simulink model "CoupledTanks_original"  (R2023b)
settings: Solver=ode45  StartTime=0.0  StopTime=400  MaxStep=1e-1  RelTol=1e-3  EnableMultiTasking=on
InitFcn:
  | g = 9.81; %gravitational constant
  | 
  | % showVR = 1; %show VR world
  | % h1_init = 0; %initial condition
  | % h2_init = 0; %initial condition
values from neighbouring files (symbols this model uses):
  K = place(Acl,Bcl, xd)    [ARI_SEM.m]
undefined symbols (not defined in the file or in its folder): P
libraries: vrlib x56, cstblocks x3, slpidlib x1
(part 2 of 2)

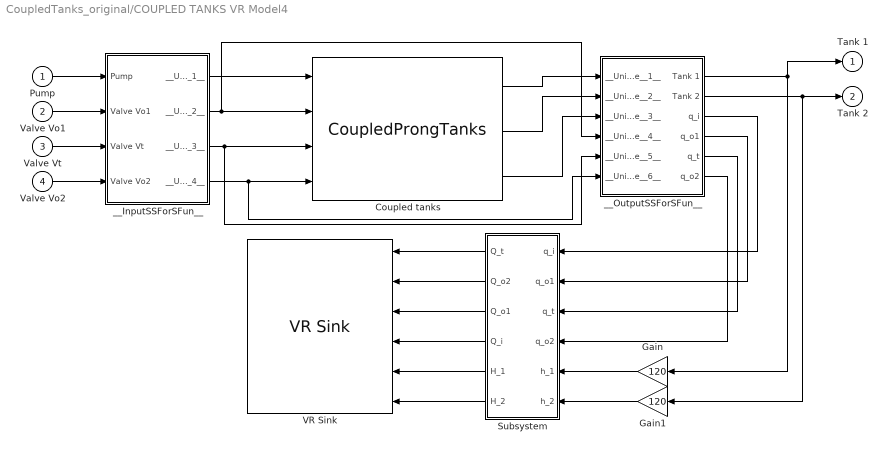
== system CoupledTanks_original/COUPLED TANKS VR Model4 ==
  Pump : Inport
  Valve Vo1 : Inport  Port=2
  Valve Vt : Inport  Port=3
  Valve Vo2 : Inport  Port=4
  Coupled tanks : M-S-Function  FunctionName=CoupledProngTanks  Parameters=h10 h20  mask{h10=sfcnParam1, h20=sfcnParam2}
      mask prompts: h10 "h1_init"; h20 "h2_init"
      mask Display:
      | port_label('input',1,'Pump');
      | port_label('input',2,'Valve Vo1');
      | port_label('input',3,'Valve Vt');
      | port_label('input',4,'Valve Vo2');
      | port_label('output',1,'Tank 1');
      | port_label('output',2,'Tank 2');
      | port_label('output',3,'q_i');
  Gain : Gain  Gain=120
  Gain1 : Gain  Gain=120
  Subsystem : Subsystem
  VR Sink : vrlib/VR Sink  InstantiateOnLoad=on  SampleTime=-1  ViewEnable=on  RemoteChange=off  RemoteView=on  FieldsWritten=Valve_t.rotation.4.1.double#Valve_o2.rotation.4.1.double#Valve_o1.rotation.4.1.double#Pump.rotation.4.1.double#water1.scale.3.1.double#water2.scale.3.1.double  WorldFileName=CoupledTanks_VR.WRL  AutoView=off  VideoDimensions=[]  AllowVariableSize=off
  __InputSSForSFun__ : Subsystem
  __OutputSSForSFun__ : Subsystem
  Tank 1 : Outport  OutDataTypeStr=double  PortDimensions=1  SampleTime=[-1 0]
  Tank 2 : Outport  Port=2  OutDataTypeStr=double  PortDimensions=1  SampleTime=[-1 0]
  wires:
  __OutputSSForSFun__/6(q_o2) -> Subsystem/4(q_o2)
  __OutputSSForSFun__/5(q_t) -> Subsystem/3(q_t)
  __OutputSSForSFun__/4(q_o1) -> Subsystem/2(q_o1)
  __OutputSSForSFun__/3(q_i) -> Subsystem/1(q_i)
  Subsystem/2(Q_o2) -> VR Sink/2
  Subsystem/3(Q_o1) -> VR Sink/3
  Subsystem/4(Q_i) -> VR Sink/4
  Subsystem/1(Q_t) -> VR Sink/1
  Subsystem/6(H_2) -> VR Sink/6
  Subsystem/5(H_1) -> VR Sink/5
  __OutputSSForSFun__/2(Tank 2) -> Gain1/1, Tank 2/1
  __OutputSSForSFun__/1(Tank 1) -> Tank 1/1, Gain/1
  __InputSSForSFun__/4(__UniqueOutportName__4__) -> __OutputSSForSFun__/6(__UniqueInportName__6__), Coupled tanks/4
  __InputSSForSFun__/3(__UniqueOutportName__3__) -> __OutputSSForSFun__/5(__UniqueInportName__5__), Coupled tanks/3
  Coupled tanks/2 -> __OutputSSForSFun__/2(__UniqueInportName__2__)
  Coupled tanks/1 -> __OutputSSForSFun__/1(__UniqueInportName__1__)
  __InputSSForSFun__/2(__UniqueOutportName__2__) -> __OutputSSForSFun__/4(__UniqueInportName__4__), Coupled tanks/2
  __InputSSForSFun__/1(__UniqueOutportName__1__) -> Coupled tanks/1
  Valve Vo2/1 -> __InputSSForSFun__/4(Valve Vo2)
  Valve Vt/1 -> __InputSSForSFun__/3(Valve Vt)
  Valve Vo1/1 -> __InputSSForSFun__/2(Valve Vo1)
  Pump/1 -> __InputSSForSFun__/1(Pump)
  Coupled tanks/3 -> __OutputSSForSFun__/3(__UniqueInportName__3__)
  Gain/1 -> Subsystem/5(h_1)
  Gain1/1 -> Subsystem/6(h_2)

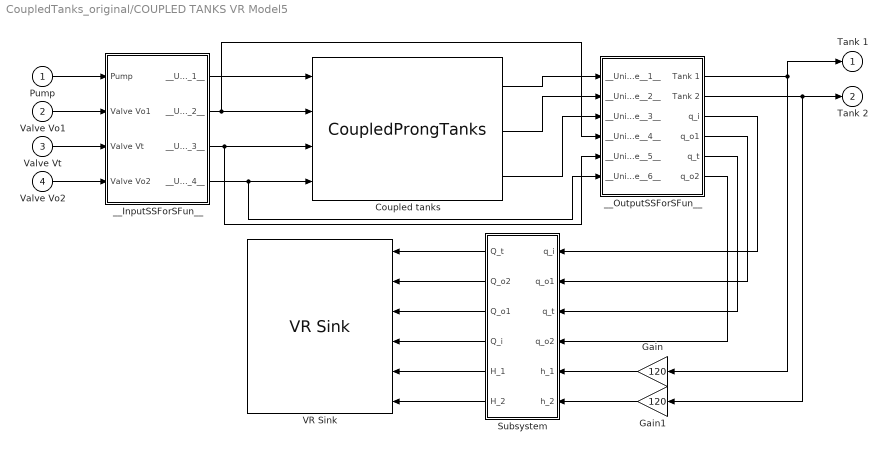
== system CoupledTanks_original/COUPLED TANKS VR Model5 ==
  Pump : Inport
  Valve Vo1 : Inport  Port=2
  Valve Vt : Inport  Port=3
  Valve Vo2 : Inport  Port=4
  Coupled tanks : M-S-Function  FunctionName=CoupledProngTanks  Parameters=h10 h20  mask{h10=sfcnParam1, h20=sfcnParam2}
      mask prompts: h10 "h1_init"; h20 "h2_init"
      mask Display:
      | port_label('input',1,'Pump');
      | port_label('input',2,'Valve Vo1');
      | port_label('input',3,'Valve Vt');
      | port_label('input',4,'Valve Vo2');
      | port_label('output',1,'Tank 1');
      | port_label('output',2,'Tank 2');
      | port_label('output',3,'q_i');
  Gain : Gain  Gain=120
  Gain1 : Gain  Gain=120
  Subsystem : Subsystem
  VR Sink : vrlib/VR Sink  InstantiateOnLoad=on  SampleTime=-1  ViewEnable=on  RemoteChange=off  RemoteView=on  FieldsWritten=Valve_t.rotation.4.1.double#Valve_o2.rotation.4.1.double#Valve_o1.rotation.4.1.double#Pump.rotation.4.1.double#water1.scale.3.1.double#water2.scale.3.1.double  WorldFileName=CoupledTanks_VR.WRL  AutoView=off  VideoDimensions=[]  AllowVariableSize=off
  __InputSSForSFun__ : Subsystem
  __OutputSSForSFun__ : Subsystem
  Tank 1 : Outport  OutDataTypeStr=double  PortDimensions=1  SampleTime=[-1 0]
  Tank 2 : Outport  Port=2  OutDataTypeStr=double  PortDimensions=1  SampleTime=[-1 0]
  wires:
  __OutputSSForSFun__/6(q_o2) -> Subsystem/4(q_o2)
  __OutputSSForSFun__/5(q_t) -> Subsystem/3(q_t)
  __OutputSSForSFun__/4(q_o1) -> Subsystem/2(q_o1)
  __OutputSSForSFun__/3(q_i) -> Subsystem/1(q_i)
  Subsystem/2(Q_o2) -> VR Sink/2
  Subsystem/3(Q_o1) -> VR Sink/3
  Subsystem/4(Q_i) -> VR Sink/4
  Subsystem/1(Q_t) -> VR Sink/1
  Subsystem/6(H_2) -> VR Sink/6
  Subsystem/5(H_1) -> VR Sink/5
  __OutputSSForSFun__/2(Tank 2) -> Gain1/1, Tank 2/1
  __OutputSSForSFun__/1(Tank 1) -> Tank 1/1, Gain/1
  __InputSSForSFun__/4(__UniqueOutportName__4__) -> __OutputSSForSFun__/6(__UniqueInportName__6__), Coupled tanks/4
  __InputSSForSFun__/3(__UniqueOutportName__3__) -> __OutputSSForSFun__/5(__UniqueInportName__5__), Coupled tanks/3
  Coupled tanks/2 -> __OutputSSForSFun__/2(__UniqueInportName__2__)
  Coupled tanks/1 -> __OutputSSForSFun__/1(__UniqueInportName__1__)
  __InputSSForSFun__/2(__UniqueOutportName__2__) -> __OutputSSForSFun__/4(__UniqueInportName__4__), Coupled tanks/2
  __InputSSForSFun__/1(__UniqueOutportName__1__) -> Coupled tanks/1
  Valve Vo2/1 -> __InputSSForSFun__/4(Valve Vo2)
  Valve Vt/1 -> __InputSSForSFun__/3(Valve Vt)
  Valve Vo1/1 -> __InputSSForSFun__/2(Valve Vo1)
  Pump/1 -> __InputSSForSFun__/1(Pump)
  Coupled tanks/3 -> __OutputSSForSFun__/3(__UniqueInportName__3__)
  Gain/1 -> Subsystem/5(h_1)
  Gain1/1 -> Subsystem/6(h_2)

== system CoupledTanks_original/COUPLED TANKS VR Model6 ==
  Pump : Inport
  Valve Vo1 : Inport  Port=2
  Valve Vt : Inport  Port=3
  Valve Vo2 : Inport  Port=4
  Coupled tanks : M-S-Function  FunctionName=CoupledProngTanks  Parameters=h10 h20  mask{h10=sfcnParam1, h20=sfcnParam2}
      mask prompts: h10 "h1_init"; h20 "h2_init"
      mask Display:
      | port_label('input',1,'Pump');
      | port_label('input',2,'Valve Vo1');
      | port_label('input',3,'Valve Vt');
      | port_label('input',4,'Valve Vo2');
      | port_label('output',1,'Tank 1');
      | port_label('output',2,'Tank 2');
      | port_label('output',3,'q_i');
  Subsystem : Subsystem
  VR Sink : vrlib/VR Sink  InstantiateOnLoad=on  SampleTime=-1  ViewEnable=on  RemoteChange=off  RemoteView=on  FieldsWritten=Valve_t.rotation.4.1.double#Valve_o2.rotation.4.1.double#Valve_o1.rotation.4.1.double#Pump.rotation.4.1.double#water1.scale.3.1.double#water2.scale.3.1.double  WorldFileName=CoupledTanks_VR.WRL  AutoView=off  VideoDimensions=[]  AllowVariableSize=off
  __InputSSForSFun__ : Subsystem
  __OutputSSForSFun__ : Subsystem
  Tank 1 : Outport  OutDataTypeStr=double  PortDimensions=1  SampleTime=[-1 0]
  Tank 2 : Outport  Port=2  OutDataTypeStr=double  PortDimensions=1  SampleTime=[-1 0]
  wires:
  __OutputSSForSFun__/6(q_o2) -> Subsystem/4(q_o2)
  __OutputSSForSFun__/5(q_t) -> Subsystem/3(q_t)
  __OutputSSForSFun__/4(q_o1) -> Subsystem/2(q_o1)
  __OutputSSForSFun__/3(q_i) -> Subsystem/1(q_i)
  Subsystem/2(Q_o2) -> VR Sink/2
  Subsystem/3(Q_o1) -> VR Sink/3
  Subsystem/4(Q_i) -> VR Sink/4
  Subsystem/1(Q_t) -> VR Sink/1
  Subsystem/6(H_2) -> VR Sink/6
  Subsystem/5(H_1) -> VR Sink/5
  __OutputSSForSFun__/2(Tank 2) -> Subsystem/6(h_2), Tank 2/1
  __OutputSSForSFun__/1(Tank 1) -> Tank 1/1, Subsystem/5(h_1)
  __InputSSForSFun__/4(__UniqueOutportName__4__) -> __OutputSSForSFun__/6(__UniqueInportName__6__), Coupled tanks/4
  __InputSSForSFun__/3(__UniqueOutportName__3__) -> __OutputSSForSFun__/5(__UniqueInportName__5__), Coupled tanks/3
  Coupled tanks/2 -> __OutputSSForSFun__/2(__UniqueInportName__2__)
  Coupled tanks/1 -> __OutputSSForSFun__/1(__UniqueInportName__1__)
  __InputSSForSFun__/2(__UniqueOutportName__2__) -> __OutputSSForSFun__/4(__UniqueInportName__4__), Coupled tanks/2
  __InputSSForSFun__/1(__UniqueOutportName__1__) -> Coupled tanks/1
  Valve Vo2/1 -> __InputSSForSFun__/4(Valve Vo2)
  Valve Vt/1 -> __InputSSForSFun__/3(Valve Vt)
  Valve Vo1/1 -> __InputSSForSFun__/2(Valve Vo1)
  Pump/1 -> __InputSSForSFun__/1(Pump)
  Coupled tanks/3 -> __OutputSSForSFun__/3(__UniqueInportName__3__)

== system CoupledTanks_original/COUPLED TANKS VR Model7 ==
  Pump : Inport
  Valve Vo1 : Inport  Port=2
  Valve Vt : Inport  Port=3
  Valve Vo2 : Inport  Port=4
  Coupled tanks : M-S-Function  FunctionName=CoupledProngTanks  Parameters=h10 h20  mask{h10=sfcnParam1, h20=sfcnParam2}
      mask prompts: h10 "h1_init"; h20 "h2_init"
      mask Display:
      | port_label('input',1,'Pump');
      | port_label('input',2,'Valve Vo1');
      | port_label('input',3,'Valve Vt');
      | port_label('input',4,'Valve Vo2');
      | port_label('output',1,'Tank 1');
      | port_label('output',2,'Tank 2');
      | port_label('output',3,'q_i');
  Gain : Gain  Gain=120
  Gain1 : Gain  Gain=120
  Subsystem : Subsystem
  VR Sink : vrlib/VR Sink  InstantiateOnLoad=on  SampleTime=-1  ViewEnable=on  RemoteChange=off  RemoteView=on  FieldsWritten=Valve_t.rotation.4.1.double#Valve_o2.rotation.4.1.double#Valve_o1.rotation.4.1.double#Pump.rotation.4.1.double#water1.scale.3.1.double#water2.scale.3.1.double  WorldFileName=CoupledTanks_VR.WRL  AutoView=off  VideoDimensions=[]  AllowVariableSize=off
  __InputSSForSFun__ : Subsystem
  __OutputSSForSFun__ : Subsystem
  Tank 1 : Outport  OutDataTypeStr=double  PortDimensions=1  SampleTime=[-1 0]
  Tank 2 : Outport  Port=2  OutDataTypeStr=double  PortDimensions=1  SampleTime=[-1 0]
  wires:
  __OutputSSForSFun__/6(q_o2) -> Subsystem/4(q_o2)
  __OutputSSForSFun__/5(q_t) -> Subsystem/3(q_t)
  __OutputSSForSFun__/4(q_o1) -> Subsystem/2(q_o1)
  __OutputSSForSFun__/3(q_i) -> Subsystem/1(q_i)
  Subsystem/2(Q_o2) -> VR Sink/2
  Subsystem/3(Q_o1) -> VR Sink/3
  Subsystem/4(Q_i) -> VR Sink/4
  Subsystem/1(Q_t) -> VR Sink/1
  Subsystem/6(H_2) -> VR Sink/6
  Subsystem/5(H_1) -> VR Sink/5
  __OutputSSForSFun__/2(Tank 2) -> Gain1/1, Tank 2/1
  __OutputSSForSFun__/1(Tank 1) -> Tank 1/1, Gain/1
  __InputSSForSFun__/4(__UniqueOutportName__4__) -> __OutputSSForSFun__/6(__UniqueInportName__6__), Coupled tanks/4
  __InputSSForSFun__/3(__UniqueOutportName__3__) -> __OutputSSForSFun__/5(__UniqueInportName__5__), Coupled tanks/3
  Coupled tanks/2 -> __OutputSSForSFun__/2(__UniqueInportName__2__)
  Coupled tanks/1 -> __OutputSSForSFun__/1(__UniqueInportName__1__)
  __InputSSForSFun__/2(__UniqueOutportName__2__) -> __OutputSSForSFun__/4(__UniqueInportName__4__), Coupled tanks/2
  __InputSSForSFun__/1(__UniqueOutportName__1__) -> Coupled tanks/1
  Valve Vo2/1 -> __InputSSForSFun__/4(Valve Vo2)
  Valve Vt/1 -> __InputSSForSFun__/3(Valve Vt)
  Valve Vo1/1 -> __InputSSForSFun__/2(Valve Vo1)
  Pump/1 -> __InputSSForSFun__/1(Pump)
  Coupled tanks/3 -> __OutputSSForSFun__/3(__UniqueInportName__3__)
  Gain/1 -> Subsystem/5(h_1)
  Gain1/1 -> Subsystem/6(h_2)

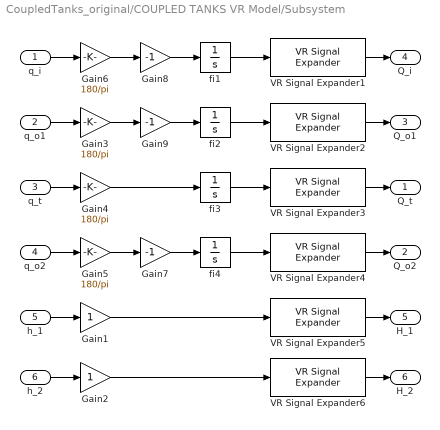
== system CoupledTanks_original/COUPLED TANKS VR Model/Subsystem ==
  q_i : Inport
  q_o1 : Inport  Port=2
  q_t : Inport  Port=3
  q_o2 : Inport  Port=4
  h_1 : Inport  Port=5
  h_2 : Inport  Port=6
  Gain1 : Gain
  Gain2 : Gain
  Gain{3..6} (4 alike) : Gain  Gain=180/pi
  Gain7 : Gain  Gain=-1
  Gain8 : Gain  Gain=-1
  Gain9 : Gain  Gain=-1
  VR Signal Expander{1..4} (4 alike) : vrlib/VR Signal Expander  outwidth=4  outidx=[4]
  VR Signal Expander5 : vrlib/VR Signal Expander  outwidth=3  outidx=[2]
  VR Signal Expander6 : vrlib/VR Signal Expander  outwidth=3  outidx=[2]
  fi{1..4} (4 alike) : Integrator
  Q_t : Outport
  Q_o2 : Outport  Port=2
  Q_o1 : Outport  Port=3
  Q_i : Outport  Port=4
  H_1 : Outport  Port=5
  H_2 : Outport  Port=6
  wires:
  Gain9/1 -> fi2/1
  Gain8/1 -> fi1/1
  Gain7/1 -> fi4/1
  Gain5/1 -> Gain7/1
  q_o2/1 -> Gain5/1
  VR Signal Expander4/1 -> Q_o2/1
  fi4/1 -> VR Signal Expander4/1
  Gain4/1 -> fi3/1
  Gain6/1 -> Gain8/1
  Gain3/1 -> Gain9/1
  q_t/1 -> Gain4/1
  q_o1/1 -> Gain3/1
  Gain2/1 -> VR Signal Expander6/1
  Gain1/1 -> VR Signal Expander5/1
  VR Signal Expander6/1 -> H_2/1
  VR Signal Expander5/1 -> H_1/1
  VR Signal Expander1/1 -> Q_i/1
  VR Signal Expander2/1 -> Q_o1/1
  VR Signal Expander3/1 -> Q_t/1
  h_2/1 -> Gain2/1
  h_1/1 -> Gain1/1
  q_i/1 -> Gain6/1
  fi2/1 -> VR Signal Expander2/1
  fi3/1 -> VR Signal Expander3/1
  fi1/1 -> VR Signal Expander1/1

== system CoupledTanks_original/COUPLED TANKS VR Model/__InputSSForSFun__ ==
  Pump : Inport
  Valve Vo1 : Inport  Port=2
  Valve Vt : Inport  Port=3
  Valve Vo2 : Inport  Port=4
  __UniqueOutportName__1__ : Outport
  __UniqueOutportName__2__ : Outport  Port=2
  __UniqueOutportName__3__ : Outport  Port=3
  __UniqueOutportName__4__ : Outport  Port=4
  wires:
  Valve Vo2/1 -> __UniqueOutportName__4__/1
  Valve Vt/1 -> __UniqueOutportName__3__/1
  Valve Vo1/1 -> __UniqueOutportName__2__/1
  Pump/1 -> __UniqueOutportName__1__/1

== system CoupledTanks_original/COUPLED TANKS VR Model/__OutputSSForSFun__ ==
  __UniqueInportName__1__ : Inport
  __UniqueInportName__2__ : Inport  Port=2
  __UniqueInportName__3__ : Inport  Port=3
  __UniqueInportName__4__ : Inport  Port=4
  __UniqueInportName__5__ : Inport  Port=5
  __UniqueInportName__6__ : Inport  Port=6
  Tank 1 : Outport  OutDataTypeStr=double  PortDimensions=1  SampleTime=[-1 0]
  Tank 2 : Outport  Port=2  OutDataTypeStr=double  PortDimensions=1  SampleTime=[-1 0]
  q_i : Outport  Port=3  OutDataTypeStr=double  PortDimensions=1  SampleTime=[0 1]
  q_o1 : Outport  Port=4  OutDataTypeStr=double  PortDimensions=1  SampleTime=[-1 0]
  q_t : Outport  Port=5  OutDataTypeStr=double  PortDimensions=1  SampleTime=[-1 0]
  q_o2 : Outport  Port=6  OutDataTypeStr=double  PortDimensions=1  SampleTime=[-1 0]
  wires:
  __UniqueInportName__6__/1 -> q_o2/1
  __UniqueInportName__5__/1 -> q_t/1
  __UniqueInportName__4__/1 -> q_o1/1
  __UniqueInportName__3__/1 -> q_i/1
  __UniqueInportName__2__/1 -> Tank 2/1
  __UniqueInportName__1__/1 -> Tank 1/1

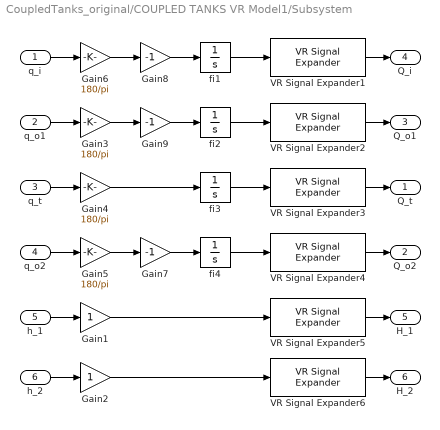
== system CoupledTanks_original/COUPLED TANKS VR Model1/Subsystem ==
  q_i : Inport
  q_o1 : Inport  Port=2
  q_t : Inport  Port=3
  q_o2 : Inport  Port=4
  h_1 : Inport  Port=5
  h_2 : Inport  Port=6
  Gain1 : Gain
  Gain2 : Gain
  Gain{3..6} (4 alike) : Gain  Gain=180/pi
  Gain7 : Gain  Gain=-1
  Gain8 : Gain  Gain=-1
  Gain9 : Gain  Gain=-1
  VR Signal Expander{1..4} (4 alike) : vrlib/VR Signal Expander  outwidth=4  outidx=[4]
  VR Signal Expander5 : vrlib/VR Signal Expander  outwidth=3  outidx=[2]
  VR Signal Expander6 : vrlib/VR Signal Expander  outwidth=3  outidx=[2]
  fi{1..4} (4 alike) : Integrator
  Q_t : Outport
  Q_o2 : Outport  Port=2
  Q_o1 : Outport  Port=3
  Q_i : Outport  Port=4
  H_1 : Outport  Port=5
  H_2 : Outport  Port=6
  wires:
  Gain9/1 -> fi2/1
  Gain8/1 -> fi1/1
  Gain7/1 -> fi4/1
  Gain5/1 -> Gain7/1
  q_o2/1 -> Gain5/1
  VR Signal Expander4/1 -> Q_o2/1
  fi4/1 -> VR Signal Expander4/1
  Gain4/1 -> fi3/1
  Gain6/1 -> Gain8/1
  Gain3/1 -> Gain9/1
  q_t/1 -> Gain4/1
  q_o1/1 -> Gain3/1
  Gain2/1 -> VR Signal Expander6/1
  Gain1/1 -> VR Signal Expander5/1
  VR Signal Expander6/1 -> H_2/1
  VR Signal Expander5/1 -> H_1/1
  VR Signal Expander1/1 -> Q_i/1
  VR Signal Expander2/1 -> Q_o1/1
  VR Signal Expander3/1 -> Q_t/1
  h_2/1 -> Gain2/1
  h_1/1 -> Gain1/1
  q_i/1 -> Gain6/1
  fi2/1 -> VR Signal Expander2/1
  fi3/1 -> VR Signal Expander3/1
  fi1/1 -> VR Signal Expander1/1

== system CoupledTanks_original/COUPLED TANKS VR Model1/__InputSSForSFun__ ==
  Pump : Inport
  Valve Vo1 : Inport  Port=2
  Valve Vt : Inport  Port=3
  Valve Vo2 : Inport  Port=4
  __UniqueOutportName__1__ : Outport
  __UniqueOutportName__2__ : Outport  Port=2
  __UniqueOutportName__3__ : Outport  Port=3
  __UniqueOutportName__4__ : Outport  Port=4
  wires:
  Valve Vo2/1 -> __UniqueOutportName__4__/1
  Valve Vt/1 -> __UniqueOutportName__3__/1
  Valve Vo1/1 -> __UniqueOutportName__2__/1
  Pump/1 -> __UniqueOutportName__1__/1

== system CoupledTanks_original/COUPLED TANKS VR Model1/__OutputSSForSFun__ ==
  __UniqueInportName__1__ : Inport
  __UniqueInportName__2__ : Inport  Port=2
  __UniqueInportName__3__ : Inport  Port=3
  __UniqueInportName__4__ : Inport  Port=4
  __UniqueInportName__5__ : Inport  Port=5
  __UniqueInportName__6__ : Inport  Port=6
  Tank 1 : Outport  OutDataTypeStr=double  PortDimensions=1  SampleTime=[-1 0]
  Tank 2 : Outport  Port=2  OutDataTypeStr=double  PortDimensions=1  SampleTime=[-1 0]
  q_i : Outport  Port=3  OutDataTypeStr=double  PortDimensions=1  SampleTime=[0 1]
  q_o1 : Outport  Port=4  OutDataTypeStr=double  PortDimensions=1  SampleTime=[-1 0]
  q_t : Outport  Port=5  OutDataTypeStr=double  PortDimensions=1  SampleTime=[-1 0]
  q_o2 : Outport  Port=6  OutDataTypeStr=double  PortDimensions=1  SampleTime=[-1 0]
  wires:
  __UniqueInportName__6__/1 -> q_o2/1
  __UniqueInportName__5__/1 -> q_t/1
  __UniqueInportName__4__/1 -> q_o1/1
  __UniqueInportName__3__/1 -> q_i/1
  __UniqueInportName__2__/1 -> Tank 2/1
  __UniqueInportName__1__/1 -> Tank 1/1

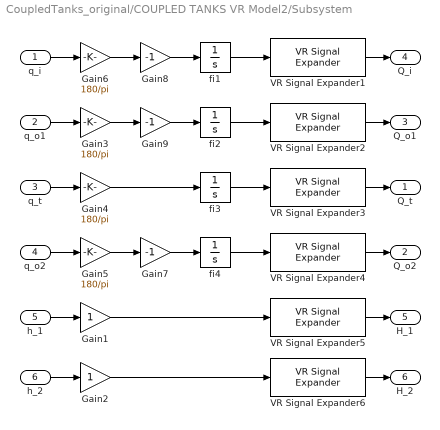
== system CoupledTanks_original/COUPLED TANKS VR Model2/Subsystem ==
  q_i : Inport
  q_o1 : Inport  Port=2
  q_t : Inport  Port=3
  q_o2 : Inport  Port=4
  h_1 : Inport  Port=5
  h_2 : Inport  Port=6
  Gain1 : Gain
  Gain2 : Gain
  Gain{3..6} (4 alike) : Gain  Gain=180/pi
  Gain7 : Gain  Gain=-1
  Gain8 : Gain  Gain=-1
  Gain9 : Gain  Gain=-1
  VR Signal Expander{1..4} (4 alike) : vrlib/VR Signal Expander  outwidth=4  outidx=[4]
  VR Signal Expander5 : vrlib/VR Signal Expander  outwidth=3  outidx=[2]
  VR Signal Expander6 : vrlib/VR Signal Expander  outwidth=3  outidx=[2]
  fi{1..4} (4 alike) : Integrator
  Q_t : Outport
  Q_o2 : Outport  Port=2
  Q_o1 : Outport  Port=3
  Q_i : Outport  Port=4
  H_1 : Outport  Port=5
  H_2 : Outport  Port=6
  wires:
  Gain9/1 -> fi2/1
  Gain8/1 -> fi1/1
  Gain7/1 -> fi4/1
  Gain5/1 -> Gain7/1
  q_o2/1 -> Gain5/1
  VR Signal Expander4/1 -> Q_o2/1
  fi4/1 -> VR Signal Expander4/1
  Gain4/1 -> fi3/1
  Gain6/1 -> Gain8/1
  Gain3/1 -> Gain9/1
  q_t/1 -> Gain4/1
  q_o1/1 -> Gain3/1
  Gain2/1 -> VR Signal Expander6/1
  Gain1/1 -> VR Signal Expander5/1
  VR Signal Expander6/1 -> H_2/1
  VR Signal Expander5/1 -> H_1/1
  VR Signal Expander1/1 -> Q_i/1
  VR Signal Expander2/1 -> Q_o1/1
  VR Signal Expander3/1 -> Q_t/1
  h_2/1 -> Gain2/1
  h_1/1 -> Gain1/1
  q_i/1 -> Gain6/1
  fi2/1 -> VR Signal Expander2/1
  fi3/1 -> VR Signal Expander3/1
  fi1/1 -> VR Signal Expander1/1

== system CoupledTanks_original/COUPLED TANKS VR Model2/__InputSSForSFun__ ==
  Pump : Inport
  Valve Vo1 : Inport  Port=2
  Valve Vt : Inport  Port=3
  Valve Vo2 : Inport  Port=4
  __UniqueOutportName__1__ : Outport
  __UniqueOutportName__2__ : Outport  Port=2
  __UniqueOutportName__3__ : Outport  Port=3
  __UniqueOutportName__4__ : Outport  Port=4
  wires:
  Valve Vo2/1 -> __UniqueOutportName__4__/1
  Valve Vt/1 -> __UniqueOutportName__3__/1
  Valve Vo1/1 -> __UniqueOutportName__2__/1
  Pump/1 -> __UniqueOutportName__1__/1

== system CoupledTanks_original/COUPLED TANKS VR Model2/__OutputSSForSFun__ ==
  __UniqueInportName__1__ : Inport
  __UniqueInportName__2__ : Inport  Port=2
  __UniqueInportName__3__ : Inport  Port=3
  __UniqueInportName__4__ : Inport  Port=4
  __UniqueInportName__5__ : Inport  Port=5
  __UniqueInportName__6__ : Inport  Port=6
  Tank 1 : Outport  OutDataTypeStr=double  PortDimensions=1  SampleTime=[-1 0]
  Tank 2 : Outport  Port=2  OutDataTypeStr=double  PortDimensions=1  SampleTime=[-1 0]
  q_i : Outport  Port=3  OutDataTypeStr=double  PortDimensions=1  SampleTime=[0 1]
  q_o1 : Outport  Port=4  OutDataTypeStr=double  PortDimensions=1  SampleTime=[-1 0]
  q_t : Outport  Port=5  OutDataTypeStr=double  PortDimensions=1  SampleTime=[-1 0]
  q_o2 : Outport  Port=6  OutDataTypeStr=double  PortDimensions=1  SampleTime=[-1 0]
  wires:
  __UniqueInportName__6__/1 -> q_o2/1
  __UniqueInportName__5__/1 -> q_t/1
  __UniqueInportName__4__/1 -> q_o1/1
  __UniqueInportName__3__/1 -> q_i/1
  __UniqueInportName__2__/1 -> Tank 2/1
  __UniqueInportName__1__/1 -> Tank 1/1

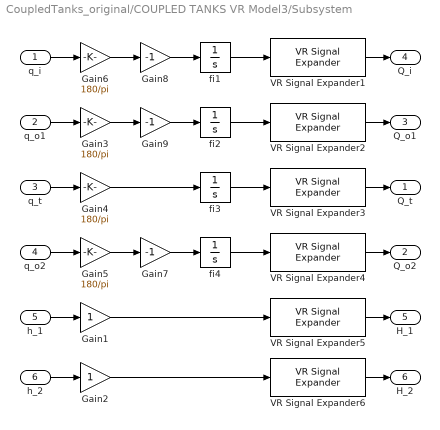
== system CoupledTanks_original/COUPLED TANKS VR Model3/Subsystem ==
  q_i : Inport
  q_o1 : Inport  Port=2
  q_t : Inport  Port=3
  q_o2 : Inport  Port=4
  h_1 : Inport  Port=5
  h_2 : Inport  Port=6
  Gain1 : Gain
  Gain2 : Gain
  Gain{3..6} (4 alike) : Gain  Gain=180/pi
  Gain7 : Gain  Gain=-1
  Gain8 : Gain  Gain=-1
  Gain9 : Gain  Gain=-1
  VR Signal Expander{1..4} (4 alike) : vrlib/VR Signal Expander  outwidth=4  outidx=[4]
  VR Signal Expander5 : vrlib/VR Signal Expander  outwidth=3  outidx=[2]
  VR Signal Expander6 : vrlib/VR Signal Expander  outwidth=3  outidx=[2]
  fi{1..4} (4 alike) : Integrator
  Q_t : Outport
  Q_o2 : Outport  Port=2
  Q_o1 : Outport  Port=3
  Q_i : Outport  Port=4
  H_1 : Outport  Port=5
  H_2 : Outport  Port=6
  wires:
  Gain9/1 -> fi2/1
  Gain8/1 -> fi1/1
  Gain7/1 -> fi4/1
  Gain5/1 -> Gain7/1
  q_o2/1 -> Gain5/1
  VR Signal Expander4/1 -> Q_o2/1
  fi4/1 -> VR Signal Expander4/1
  Gain4/1 -> fi3/1
  Gain6/1 -> Gain8/1
  Gain3/1 -> Gain9/1
  q_t/1 -> Gain4/1
  q_o1/1 -> Gain3/1
  Gain2/1 -> VR Signal Expander6/1
  Gain1/1 -> VR Signal Expander5/1
  VR Signal Expander6/1 -> H_2/1
  VR Signal Expander5/1 -> H_1/1
  VR Signal Expander1/1 -> Q_i/1
  VR Signal Expander2/1 -> Q_o1/1
  VR Signal Expander3/1 -> Q_t/1
  h_2/1 -> Gain2/1
  h_1/1 -> Gain1/1
  q_i/1 -> Gain6/1
  fi2/1 -> VR Signal Expander2/1
  fi3/1 -> VR Signal Expander3/1
  fi1/1 -> VR Signal Expander1/1

== system CoupledTanks_original/COUPLED TANKS VR Model3/__InputSSForSFun__ ==
  Pump : Inport
  Valve Vo1 : Inport  Port=2
  Valve Vt : Inport  Port=3
  Valve Vo2 : Inport  Port=4
  __UniqueOutportName__1__ : Outport
  __UniqueOutportName__2__ : Outport  Port=2
  __UniqueOutportName__3__ : Outport  Port=3
  __UniqueOutportName__4__ : Outport  Port=4
  wires:
  Valve Vo2/1 -> __UniqueOutportName__4__/1
  Valve Vt/1 -> __UniqueOutportName__3__/1
  Valve Vo1/1 -> __UniqueOutportName__2__/1
  Pump/1 -> __UniqueOutportName__1__/1

== system CoupledTanks_original/COUPLED TANKS VR Model3/__OutputSSForSFun__ ==
  __UniqueInportName__1__ : Inport
  __UniqueInportName__2__ : Inport  Port=2
  __UniqueInportName__3__ : Inport  Port=3
  __UniqueInportName__4__ : Inport  Port=4
  __UniqueInportName__5__ : Inport  Port=5
  __UniqueInportName__6__ : Inport  Port=6
  Tank 1 : Outport  OutDataTypeStr=double  PortDimensions=1  SampleTime=[-1 0]
  Tank 2 : Outport  Port=2  OutDataTypeStr=double  PortDimensions=1  SampleTime=[-1 0]
  q_i : Outport  Port=3  OutDataTypeStr=double  PortDimensions=1  SampleTime=[0 1]
  q_o1 : Outport  Port=4  OutDataTypeStr=double  PortDimensions=1  SampleTime=[-1 0]
  q_t : Outport  Port=5  OutDataTypeStr=double  PortDimensions=1  SampleTime=[-1 0]
  q_o2 : Outport  Port=6  OutDataTypeStr=double  PortDimensions=1  SampleTime=[-1 0]
  wires:
  __UniqueInportName__6__/1 -> q_o2/1
  __UniqueInportName__5__/1 -> q_t/1
  __UniqueInportName__4__/1 -> q_o1/1
  __UniqueInportName__3__/1 -> q_i/1
  __UniqueInportName__2__/1 -> Tank 2/1
  __UniqueInportName__1__/1 -> Tank 1/1

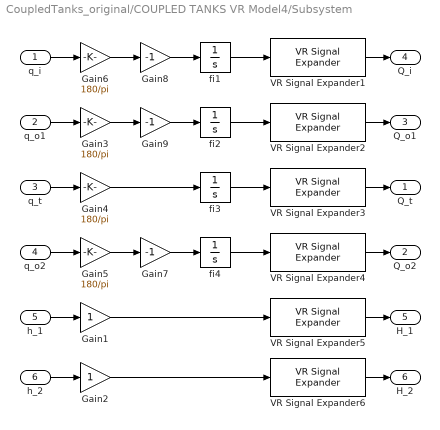
== system CoupledTanks_original/COUPLED TANKS VR Model4/Subsystem ==
  q_i : Inport
  q_o1 : Inport  Port=2
  q_t : Inport  Port=3
  q_o2 : Inport  Port=4
  h_1 : Inport  Port=5
  h_2 : Inport  Port=6
  Gain1 : Gain
  Gain2 : Gain
  Gain{3..6} (4 alike) : Gain  Gain=180/pi
  Gain7 : Gain  Gain=-1
  Gain8 : Gain  Gain=-1
  Gain9 : Gain  Gain=-1
  VR Signal Expander{1..4} (4 alike) : vrlib/VR Signal Expander  outwidth=4  outidx=[4]
  VR Signal Expander5 : vrlib/VR Signal Expander  outwidth=3  outidx=[2]
  VR Signal Expander6 : vrlib/VR Signal Expander  outwidth=3  outidx=[2]
  fi{1..4} (4 alike) : Integrator
  Q_t : Outport
  Q_o2 : Outport  Port=2
  Q_o1 : Outport  Port=3
  Q_i : Outport  Port=4
  H_1 : Outport  Port=5
  H_2 : Outport  Port=6
  wires:
  Gain9/1 -> fi2/1
  Gain8/1 -> fi1/1
  Gain7/1 -> fi4/1
  Gain5/1 -> Gain7/1
  q_o2/1 -> Gain5/1
  VR Signal Expander4/1 -> Q_o2/1
  fi4/1 -> VR Signal Expander4/1
  Gain4/1 -> fi3/1
  Gain6/1 -> Gain8/1
  Gain3/1 -> Gain9/1
  q_t/1 -> Gain4/1
  q_o1/1 -> Gain3/1
  Gain2/1 -> VR Signal Expander6/1
  Gain1/1 -> VR Signal Expander5/1
  VR Signal Expander6/1 -> H_2/1
  VR Signal Expander5/1 -> H_1/1
  VR Signal Expander1/1 -> Q_i/1
  VR Signal Expander2/1 -> Q_o1/1
  VR Signal Expander3/1 -> Q_t/1
  h_2/1 -> Gain2/1
  h_1/1 -> Gain1/1
  q_i/1 -> Gain6/1
  fi2/1 -> VR Signal Expander2/1
  fi3/1 -> VR Signal Expander3/1
  fi1/1 -> VR Signal Expander1/1

== system CoupledTanks_original/COUPLED TANKS VR Model4/__InputSSForSFun__ ==
  Pump : Inport
  Valve Vo1 : Inport  Port=2
  Valve Vt : Inport  Port=3
  Valve Vo2 : Inport  Port=4
  __UniqueOutportName__1__ : Outport
  __UniqueOutportName__2__ : Outport  Port=2
  __UniqueOutportName__3__ : Outport  Port=3
  __UniqueOutportName__4__ : Outport  Port=4
  wires:
  Valve Vo2/1 -> __UniqueOutportName__4__/1
  Valve Vt/1 -> __UniqueOutportName__3__/1
  Valve Vo1/1 -> __UniqueOutportName__2__/1
  Pump/1 -> __UniqueOutportName__1__/1

== system CoupledTanks_original/COUPLED TANKS VR Model4/__OutputSSForSFun__ ==
  __UniqueInportName__1__ : Inport
  __UniqueInportName__2__ : Inport  Port=2
  __UniqueInportName__3__ : Inport  Port=3
  __UniqueInportName__4__ : Inport  Port=4
  __UniqueInportName__5__ : Inport  Port=5
  __UniqueInportName__6__ : Inport  Port=6
  Tank 1 : Outport  OutDataTypeStr=double  PortDimensions=1  SampleTime=[-1 0]
  Tank 2 : Outport  Port=2  OutDataTypeStr=double  PortDimensions=1  SampleTime=[-1 0]
  q_i : Outport  Port=3  OutDataTypeStr=double  PortDimensions=1  SampleTime=[0 1]
  q_o1 : Outport  Port=4  OutDataTypeStr=double  PortDimensions=1  SampleTime=[-1 0]
  q_t : Outport  Port=5  OutDataTypeStr=double  PortDimensions=1  SampleTime=[-1 0]
  q_o2 : Outport  Port=6  OutDataTypeStr=double  PortDimensions=1  SampleTime=[-1 0]
  wires:
  __UniqueInportName__6__/1 -> q_o2/1
  __UniqueInportName__5__/1 -> q_t/1
  __UniqueInportName__4__/1 -> q_o1/1
  __UniqueInportName__3__/1 -> q_i/1
  __UniqueInportName__2__/1 -> Tank 2/1
  __UniqueInportName__1__/1 -> Tank 1/1

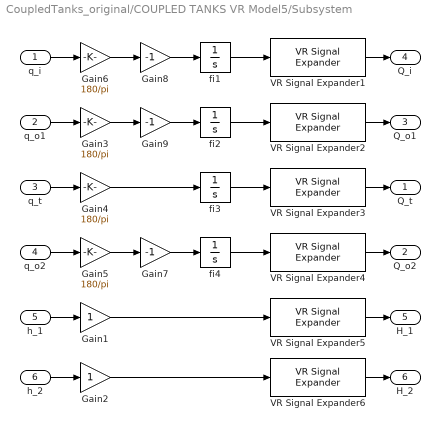
== system CoupledTanks_original/COUPLED TANKS VR Model5/Subsystem ==
  q_i : Inport
  q_o1 : Inport  Port=2
  q_t : Inport  Port=3
  q_o2 : Inport  Port=4
  h_1 : Inport  Port=5
  h_2 : Inport  Port=6
  Gain1 : Gain
  Gain2 : Gain
  Gain{3..6} (4 alike) : Gain  Gain=180/pi
  Gain7 : Gain  Gain=-1
  Gain8 : Gain  Gain=-1
  Gain9 : Gain  Gain=-1
  VR Signal Expander{1..4} (4 alike) : vrlib/VR Signal Expander  outwidth=4  outidx=[4]
  VR Signal Expander5 : vrlib/VR Signal Expander  outwidth=3  outidx=[2]
  VR Signal Expander6 : vrlib/VR Signal Expander  outwidth=3  outidx=[2]
  fi{1..4} (4 alike) : Integrator
  Q_t : Outport
  Q_o2 : Outport  Port=2
  Q_o1 : Outport  Port=3
  Q_i : Outport  Port=4
  H_1 : Outport  Port=5
  H_2 : Outport  Port=6
  wires:
  Gain9/1 -> fi2/1
  Gain8/1 -> fi1/1
  Gain7/1 -> fi4/1
  Gain5/1 -> Gain7/1
  q_o2/1 -> Gain5/1
  VR Signal Expander4/1 -> Q_o2/1
  fi4/1 -> VR Signal Expander4/1
  Gain4/1 -> fi3/1
  Gain6/1 -> Gain8/1
  Gain3/1 -> Gain9/1
  q_t/1 -> Gain4/1
  q_o1/1 -> Gain3/1
  Gain2/1 -> VR Signal Expander6/1
  Gain1/1 -> VR Signal Expander5/1
  VR Signal Expander6/1 -> H_2/1
  VR Signal Expander5/1 -> H_1/1
  VR Signal Expander1/1 -> Q_i/1
  VR Signal Expander2/1 -> Q_o1/1
  VR Signal Expander3/1 -> Q_t/1
  h_2/1 -> Gain2/1
  h_1/1 -> Gain1/1
  q_i/1 -> Gain6/1
  fi2/1 -> VR Signal Expander2/1
  fi3/1 -> VR Signal Expander3/1
  fi1/1 -> VR Signal Expander1/1

== system CoupledTanks_original/COUPLED TANKS VR Model5/__InputSSForSFun__ ==
  Pump : Inport
  Valve Vo1 : Inport  Port=2
  Valve Vt : Inport  Port=3
  Valve Vo2 : Inport  Port=4
  __UniqueOutportName__1__ : Outport
  __UniqueOutportName__2__ : Outport  Port=2
  __UniqueOutportName__3__ : Outport  Port=3
  __UniqueOutportName__4__ : Outport  Port=4
  wires:
  Valve Vo2/1 -> __UniqueOutportName__4__/1
  Valve Vt/1 -> __UniqueOutportName__3__/1
  Valve Vo1/1 -> __UniqueOutportName__2__/1
  Pump/1 -> __UniqueOutportName__1__/1

== system CoupledTanks_original/COUPLED TANKS VR Model5/__OutputSSForSFun__ ==
  __UniqueInportName__1__ : Inport
  __UniqueInportName__2__ : Inport  Port=2
  __UniqueInportName__3__ : Inport  Port=3
  __UniqueInportName__4__ : Inport  Port=4
  __UniqueInportName__5__ : Inport  Port=5
  __UniqueInportName__6__ : Inport  Port=6
  Tank 1 : Outport  OutDataTypeStr=double  PortDimensions=1  SampleTime=[-1 0]
  Tank 2 : Outport  Port=2  OutDataTypeStr=double  PortDimensions=1  SampleTime=[-1 0]
  q_i : Outport  Port=3  OutDataTypeStr=double  PortDimensions=1  SampleTime=[0 1]
  q_o1 : Outport  Port=4  OutDataTypeStr=double  PortDimensions=1  SampleTime=[-1 0]
  q_t : Outport  Port=5  OutDataTypeStr=double  PortDimensions=1  SampleTime=[-1 0]
  q_o2 : Outport  Port=6  OutDataTypeStr=double  PortDimensions=1  SampleTime=[-1 0]
  wires:
  __UniqueInportName__6__/1 -> q_o2/1
  __UniqueInportName__5__/1 -> q_t/1
  __UniqueInportName__4__/1 -> q_o1/1
  __UniqueInportName__3__/1 -> q_i/1
  __UniqueInportName__2__/1 -> Tank 2/1
  __UniqueInportName__1__/1 -> Tank 1/1

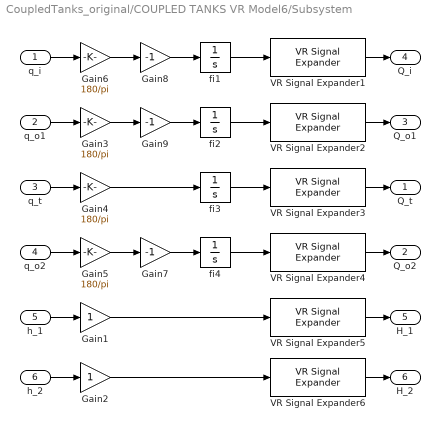
== system CoupledTanks_original/COUPLED TANKS VR Model6/Subsystem ==
  q_i : Inport
  q_o1 : Inport  Port=2
  q_t : Inport  Port=3
  q_o2 : Inport  Port=4
  h_1 : Inport  Port=5
  h_2 : Inport  Port=6
  Gain1 : Gain
  Gain2 : Gain
  Gain{3..6} (4 alike) : Gain  Gain=180/pi
  Gain7 : Gain  Gain=-1
  Gain8 : Gain  Gain=-1
  Gain9 : Gain  Gain=-1
  VR Signal Expander{1..4} (4 alike) : vrlib/VR Signal Expander  outwidth=4  outidx=[4]
  VR Signal Expander5 : vrlib/VR Signal Expander  outwidth=3  outidx=[2]
  VR Signal Expander6 : vrlib/VR Signal Expander  outwidth=3  outidx=[2]
  fi{1..4} (4 alike) : Integrator
  Q_t : Outport
  Q_o2 : Outport  Port=2
  Q_o1 : Outport  Port=3
  Q_i : Outport  Port=4
  H_1 : Outport  Port=5
  H_2 : Outport  Port=6
  wires:
  Gain9/1 -> fi2/1
  Gain8/1 -> fi1/1
  Gain7/1 -> fi4/1
  Gain5/1 -> Gain7/1
  q_o2/1 -> Gain5/1
  VR Signal Expander4/1 -> Q_o2/1
  fi4/1 -> VR Signal Expander4/1
  Gain4/1 -> fi3/1
  Gain6/1 -> Gain8/1
  Gain3/1 -> Gain9/1
  q_t/1 -> Gain4/1
  q_o1/1 -> Gain3/1
  Gain2/1 -> VR Signal Expander6/1
  Gain1/1 -> VR Signal Expander5/1
  VR Signal Expander6/1 -> H_2/1
  VR Signal Expander5/1 -> H_1/1
  VR Signal Expander1/1 -> Q_i/1
  VR Signal Expander2/1 -> Q_o1/1
  VR Signal Expander3/1 -> Q_t/1
  h_2/1 -> Gain2/1
  h_1/1 -> Gain1/1
  q_i/1 -> Gain6/1
  fi2/1 -> VR Signal Expander2/1
  fi3/1 -> VR Signal Expander3/1
  fi1/1 -> VR Signal Expander1/1

== system CoupledTanks_original/COUPLED TANKS VR Model6/__InputSSForSFun__ ==
  Pump : Inport
  Valve Vo1 : Inport  Port=2
  Valve Vt : Inport  Port=3
  Valve Vo2 : Inport  Port=4
  __UniqueOutportName__1__ : Outport
  __UniqueOutportName__2__ : Outport  Port=2
  __UniqueOutportName__3__ : Outport  Port=3
  __UniqueOutportName__4__ : Outport  Port=4
  wires:
  Valve Vo2/1 -> __UniqueOutportName__4__/1
  Valve Vt/1 -> __UniqueOutportName__3__/1
  Valve Vo1/1 -> __UniqueOutportName__2__/1
  Pump/1 -> __UniqueOutportName__1__/1

== system CoupledTanks_original/COUPLED TANKS VR Model6/__OutputSSForSFun__ ==
  __UniqueInportName__1__ : Inport
  __UniqueInportName__2__ : Inport  Port=2
  __UniqueInportName__3__ : Inport  Port=3
  __UniqueInportName__4__ : Inport  Port=4
  __UniqueInportName__5__ : Inport  Port=5
  __UniqueInportName__6__ : Inport  Port=6
  Tank 1 : Outport  OutDataTypeStr=double  PortDimensions=1  SampleTime=[-1 0]
  Tank 2 : Outport  Port=2  OutDataTypeStr=double  PortDimensions=1  SampleTime=[-1 0]
  q_i : Outport  Port=3  OutDataTypeStr=double  PortDimensions=1  SampleTime=[0 1]
  q_o1 : Outport  Port=4  OutDataTypeStr=double  PortDimensions=1  SampleTime=[-1 0]
  q_t : Outport  Port=5  OutDataTypeStr=double  PortDimensions=1  SampleTime=[-1 0]
  q_o2 : Outport  Port=6  OutDataTypeStr=double  PortDimensions=1  SampleTime=[-1 0]
  wires:
  __UniqueInportName__6__/1 -> q_o2/1
  __UniqueInportName__5__/1 -> q_t/1
  __UniqueInportName__4__/1 -> q_o1/1
  __UniqueInportName__3__/1 -> q_i/1
  __UniqueInportName__2__/1 -> Tank 2/1
  __UniqueInportName__1__/1 -> Tank 1/1

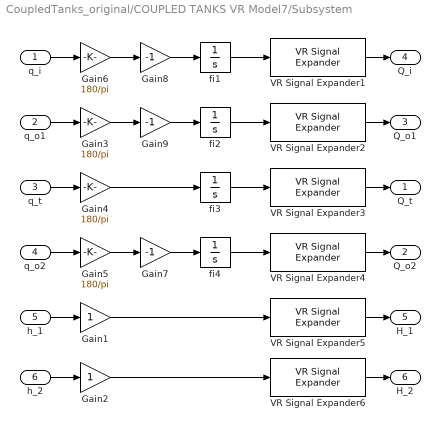
== system CoupledTanks_original/COUPLED TANKS VR Model7/Subsystem ==
  q_i : Inport
  q_o1 : Inport  Port=2
  q_t : Inport  Port=3
  q_o2 : Inport  Port=4
  h_1 : Inport  Port=5
  h_2 : Inport  Port=6
  Gain1 : Gain
  Gain2 : Gain
  Gain{3..6} (4 alike) : Gain  Gain=180/pi
  Gain7 : Gain  Gain=-1
  Gain8 : Gain  Gain=-1
  Gain9 : Gain  Gain=-1
  VR Signal Expander{1..4} (4 alike) : vrlib/VR Signal Expander  outwidth=4  outidx=[4]
  VR Signal Expander5 : vrlib/VR Signal Expander  outwidth=3  outidx=[2]
  VR Signal Expander6 : vrlib/VR Signal Expander  outwidth=3  outidx=[2]
  fi{1..4} (4 alike) : Integrator
  Q_t : Outport
  Q_o2 : Outport  Port=2
  Q_o1 : Outport  Port=3
  Q_i : Outport  Port=4
  H_1 : Outport  Port=5
  H_2 : Outport  Port=6
  wires:
  Gain9/1 -> fi2/1
  Gain8/1 -> fi1/1
  Gain7/1 -> fi4/1
  Gain5/1 -> Gain7/1
  q_o2/1 -> Gain5/1
  VR Signal Expander4/1 -> Q_o2/1
  fi4/1 -> VR Signal Expander4/1
  Gain4/1 -> fi3/1
  Gain6/1 -> Gain8/1
  Gain3/1 -> Gain9/1
  q_t/1 -> Gain4/1
  q_o1/1 -> Gain3/1
  Gain2/1 -> VR Signal Expander6/1
  Gain1/1 -> VR Signal Expander5/1
  VR Signal Expander6/1 -> H_2/1
  VR Signal Expander5/1 -> H_1/1
  VR Signal Expander1/1 -> Q_i/1
  VR Signal Expander2/1 -> Q_o1/1
  VR Signal Expander3/1 -> Q_t/1
  h_2/1 -> Gain2/1
  h_1/1 -> Gain1/1
  q_i/1 -> Gain6/1
  fi2/1 -> VR Signal Expander2/1
  fi3/1 -> VR Signal Expander3/1
  fi1/1 -> VR Signal Expander1/1

== system CoupledTanks_original/COUPLED TANKS VR Model7/__InputSSForSFun__ ==
  Pump : Inport
  Valve Vo1 : Inport  Port=2
  Valve Vt : Inport  Port=3
  Valve Vo2 : Inport  Port=4
  __UniqueOutportName__1__ : Outport
  __UniqueOutportName__2__ : Outport  Port=2
  __UniqueOutportName__3__ : Outport  Port=3
  __UniqueOutportName__4__ : Outport  Port=4
  wires:
  Valve Vo2/1 -> __UniqueOutportName__4__/1
  Valve Vt/1 -> __UniqueOutportName__3__/1
  Valve Vo1/1 -> __UniqueOutportName__2__/1
  Pump/1 -> __UniqueOutportName__1__/1

== system CoupledTanks_original/COUPLED TANKS VR Model7/__OutputSSForSFun__ ==
  __UniqueInportName__1__ : Inport
  __UniqueInportName__2__ : Inport  Port=2
  __UniqueInportName__3__ : Inport  Port=3
  __UniqueInportName__4__ : Inport  Port=4
  __UniqueInportName__5__ : Inport  Port=5
  __UniqueInportName__6__ : Inport  Port=6
  Tank 1 : Outport  OutDataTypeStr=double  PortDimensions=1  SampleTime=[-1 0]
  Tank 2 : Outport  Port=2  OutDataTypeStr=double  PortDimensions=1  SampleTime=[-1 0]
  q_i : Outport  Port=3  OutDataTypeStr=double  PortDimensions=1  SampleTime=[0 1]
  q_o1 : Outport  Port=4  OutDataTypeStr=double  PortDimensions=1  SampleTime=[-1 0]
  q_t : Outport  Port=5  OutDataTypeStr=double  PortDimensions=1  SampleTime=[-1 0]
  q_o2 : Outport  Port=6  OutDataTypeStr=double  PortDimensions=1  SampleTime=[-1 0]
  wires:
  __UniqueInportName__6__/1 -> q_o2/1
  __UniqueInportName__5__/1 -> q_t/1
  __UniqueInportName__4__/1 -> q_o1/1
  __UniqueInportName__3__/1 -> q_i/1
  __UniqueInportName__2__/1 -> Tank 2/1
  __UniqueInportName__1__/1 -> Tank 1/1
